simulink model "eVTOL_PX4_2023b"  (R2024b)
settings: Solver=ode4  StartTime=0  StopTime=inf  FixedStep=0.01  RelTol=1e-3
values from neighbouring files (symbols this model uses):
  aDl =     [initdata.mat]
  aDr =     [initdata.mat]
  aDyn =     [initdata.mat]
  Airport = init_airport('PHNL')    [initdata_HIL_eVTOL.m]
  aLat =     [initdata.mat]
  aLon =     [initdata.mat]
  D = Prop.D    [EOM_dt_MC.m]    (also in EOM_get_alf_dt_de_prop_evtol.m = CD * QS)
  dt0 = X(2)    [EOM_get_alf_dt_de_prop_evtol.m]    (also in initdata.mat = 0.258252593971; initdata_HIL_eVTOL.m = EOM_dt_MC)
  EAS0 = TAS0 / EAS2TAS    [initdata_HIL_eVTOL.m]
  FCS = init_FCS    [initdata_HIL_eVTOL.m]
  General = init_layoutdata    [EOM_dt_MC.m]    (also in build_optimized_CA.m; initdata.mat = ; initdata_HIL_eVTOL.m)
  h0 = Con(1)    [EOM_get_alf_dt_de_prop_evtol.m]    (also in initdata.mat = 450; initdata_HIL_eVTOL.m = 50)
  mass = Con(3)    [EOM_get_alf_dt_de_prop_evtol.m]    (also in initdata.mat = 2255.54; initdata_HIL_eVTOL.m = 7)
  Motor = init_motor_evtol    [EOM_dt_MC.m]    (also in initdata.mat = []; initdata_HIL_eVTOL.m)
  Prop = init_propeller_evtol_new    [EOM_dt_MC.m]    (also in initdata_HIL_eVTOL.m)
  R2D = 180/pi    (= 57.2957795131)    [EOM_get_alf_dt_de_prop_evtol.m]    (also in init_FCS.m; init_aerodata_evtol.m; init_airport.m; initdata.mat)
  SAMPLE_TIME = 0.01    [initdata_HIL_eVTOL.m]
  theta0 = -0.0510981441662    [initdata.mat]
undefined symbols (not defined in the file or in its folder): A1, aDa, aDe, aero, asbhl20env, B1, C1, de0, Earth, Environment, INIT_Data, InitData, Kd, Kp, magnitude, Newton, pProp, Raphson, Tc, WGS84
libraries: simulink_extras x63, vrlib x48, sharedtransform x28, simulink x22, slpidlib x20, sharedutil x20, matrix_library x18, aerolibwindfilters x12, aerolibobsolete x8, aerolibasang x8, aerolibatmos2 x6, aerolibfltsims x6
(part 15 of 17)

== system eVTOL_PX4_2023b/Subsystem1/Environment1/Wind Models/Dryden Wind Turbulence Model (Continuous (+q -r))/Select angular rates/Medium//High altitude rates ==
  pgw_h&l : Inport
  qgw_h&l : Inport  Port=2
  rgw_h&l : Inport  Port=3
  Action Port : ActionPort  PropagateVarSize=During execution  ActionPortLabel=elseif(u1>=min_height_high)
  Gain : Gain  SaturateOnIntegerOverflow=on  OutDataTypeStr=Inherit: Same as input  ParamDataTypeStr=Inherit: Same as input
  Mux : Mux  Inputs=3
  Selector3 : Selector  InputPortWidth=6  IndexOptions=Index vector (dialog)  Indices=[ 2 4 6]  OutputSizes=1
  pgw,qgw,rgw : Outport  InitialOutput=0  VectorParamsAs1DForOutWhenUnconnected=off
  wires:
  Gain/1 -> pgw,qgw,rgw/1
  Selector3/1 -> Gain/1
  pgw_h&l/1 -> Mux/1
  qgw_h&l/1 -> Mux/2
  rgw_h&l/1 -> Mux/3
  Mux/1 -> Selector3/1

== system eVTOL_PX4_2023b/Subsystem1/Environment1/Wind Models/Dryden Wind Turbulence Model (Continuous (+q -r))/Select angular rates/Merge Subsystems ==
  low : Inport
  high : Inport  Port=2
  interpolated : Inport  Port=3
  Demux : Demux  Outputs=3
      settings: DisplayOption=none
  Merge : Merge  Inputs=3
  pgw : Outport  VectorParamsAs1DForOutWhenUnconnected=off
  qgw : Outport  Port=2  VectorParamsAs1DForOutWhenUnconnected=off
  rgw : Outport  Port=3  VectorParamsAs1DForOutWhenUnconnected=off
  wires:
  low/1 -> Merge/1
  high/1 -> Merge/2
  interpolated/1 -> Merge/3
  Demux/2 -> qgw/1
  Demux/3 -> rgw/1
  Demux/1 -> pgw/1
  Merge/1 -> Demux/1

== system eVTOL_PX4_2023b/Subsystem1/Environment1/Wind Models/Dryden Wind Turbulence Model (Continuous (+q -r))/Select velocities/Interpolate velocities ==
  ugw_h&l : Inport
  vgw_h&l : Inport  Port=2
  wgw_h&l : Inport  Port=3
  DCM : Inport  Port=4
  Wind direction : Inport  Port=5
  Altitude : Inport  Port=6
  Action Port : ActionPort  PropagateVarSize=During execution  ActionPortLabel=else
  Mux : Mux  Inputs=3
  Mux1 : Mux  Inputs=3
  Product1 : Product  Inputs=**/  SaturateOnIntegerOverflow=on  OutDataTypeStr=Inherit: Same as first input
  Selector : Selector  InputPortWidth=2  IndexOptions=Index vector (dialog)  Indices=1  OutputSizes=1
  Selector1 : Selector  InputPortWidth=2  IndexOptions=Index vector (dialog)  Indices=1  OutputSizes=1
  Selector2 : Selector  InputPortWidth=2  IndexOptions=Index vector (dialog)  Indices=1  OutputSizes=1
  Selector3 : Selector  InputPortWidth=2  IndexOptions=Index vector (dialog)  Indices=2  OutputSizes=1
  Selector4 : Selector  InputPortWidth=2  IndexOptions=Index vector (dialog)  Indices=2  OutputSizes=1
  Selector5 : Selector  InputPortWidth=2  IndexOptions=Index vector (dialog)  Indices=2  OutputSizes=1
  Sum : Sum  Inputs=|-+  SaturateOnIntegerOverflow=on
  Sum1 : Sum  Inputs=|+-  SaturateOnIntegerOverflow=on
  Sum2 : Sum  Inputs=-+|  SaturateOnIntegerOverflow=on
  Sum3 : Sum  Inputs=++|  SaturateOnIntegerOverflow=on
  max_height_low : Constant  Value=max_height_low
  min_height_high : Constant  Value=min_height_high
  wind to body transformation : Subsystem
  ugw,vgw,wgw : Outport  InitialOutput=0  VectorParamsAs1DForOutWhenUnconnected=off
  wires:
  Mux/1 -> wind to body transformation/3(ug_l,vg_l,wg_l)
  Wind direction/1 -> wind to body transformation/2(Wind direction)
  DCM/1 -> wind to body transformation/1(DCM)
  wind to body transformation/1(ug,vg,wg) -> Sum3/1, Sum2/1
  Sum3/1 -> ugw,vgw,wgw/1
  Product1/1 -> Sum3/2
  Mux1/1 -> Sum2/2
  Sum2/1 -> Product1/1
  Sum1/1 -> Product1/2
  Sum/1 -> Product1/3
  Altitude/1 -> Sum1/1
  min_height_high/1 -> Sum/2
  max_height_low/1 -> Sum1/2, Sum/1
  Selector3/1 -> Mux1/1
  Selector4/1 -> Mux1/2
  Selector5/1 -> Mux1/3
  ugw_h&l/1 -> Selector/1, Selector3/1
  vgw_h&l/1 -> Selector4/1, Selector1/1
  wgw_h&l/1 -> Selector5/1, Selector2/1
  Selector/1 -> Mux/1
  Selector1/1 -> Mux/2
  Selector2/1 -> Mux/3

== system eVTOL_PX4_2023b/Subsystem1/Environment1/Wind Models/Dryden Wind Turbulence Model (Continuous (+q -r))/Select velocities/Low altitude velocities ==
  DCM : Inport
  ugw_h&l : Inport  Port=2
  vgw_h&l : Inport  Port=3
  wgw_h&l : Inport  Port=4
  Wind direction : Inport  Port=5
  Action Port : ActionPort  PropagateVarSize=During execution  ActionPortLabel=if(u1<=max_height_low)
  Mux : Mux  Inputs=3
  Selector : Selector  InputPortWidth=2  IndexOptions=Index vector (dialog)  Indices=1  OutputSizes=1
  Selector1 : Selector  InputPortWidth=2  IndexOptions=Index vector (dialog)  Indices=1  OutputSizes=1
  Selector2 : Selector  InputPortWidth=2  IndexOptions=Index vector (dialog)  Indices=1  OutputSizes=1
  wind to body transformation : Subsystem
  ugw,vgw,wgw : Outport  InitialOutput=0  VectorParamsAs1DForOutWhenUnconnected=off
  wires:
  Mux/1 -> wind to body transformation/3(ug_l,vg_l,wg_l)
  Selector2/1 -> Mux/3
  wind to body transformation/1(ug,vg,wg) -> ugw,vgw,wgw/1
  Wind direction/1 -> wind to body transformation/2(Wind direction)
  DCM/1 -> wind to body transformation/1(DCM)
  Selector1/1 -> Mux/2
  Selector/1 -> Mux/1
  wgw_h&l/1 -> Selector2/1
  vgw_h&l/1 -> Selector1/1
  ugw_h&l/1 -> Selector/1

== system eVTOL_PX4_2023b/Subsystem1/Environment1/Wind Models/Dryden Wind Turbulence Model (Continuous (+q -r))/Select velocities/Medium//High altitude velocities ==
  ugw_h&l : Inport
  vgw_h&l : Inport  Port=2
  wgw_h&l : Inport  Port=3
  Action Port : ActionPort  PropagateVarSize=During execution  ActionPortLabel=elseif(u1>=min_height_high)
  Gain : Gain  SaturateOnIntegerOverflow=on  OutDataTypeStr=Inherit: Same as input  ParamDataTypeStr=Inherit: Same as input
  Mux : Mux  Inputs=3
  Selector3 : Selector  InputPortWidth=6  IndexOptions=Index vector (dialog)  Indices=[ 2 4 6]  OutputSizes=1
  ugw,vgw,wgw : Outport  InitialOutput=0  VectorParamsAs1DForOutWhenUnconnected=off
  wires:
  vgw_h&l/1 -> Mux/2
  Gain/1 -> ugw,vgw,wgw/1
  Selector3/1 -> Gain/1
  Mux/1 -> Selector3/1
  wgw_h&l/1 -> Mux/3
  ugw_h&l/1 -> Mux/1

== system eVTOL_PX4_2023b/Subsystem1/Environment1/Wind Models/Dryden Wind Turbulence Model (Continuous (+q -r))/Select velocities/Merge Subsystems ==
  low : Inport
  high : Inport  Port=2
  interpolated : Inport  Port=3
  Demux : Demux  Outputs=3
      settings: DisplayOption=none
  Merge : Merge  Inputs=3
  ugw : Outport  VectorParamsAs1DForOutWhenUnconnected=off
  vgw : Outport  Port=2  VectorParamsAs1DForOutWhenUnconnected=off
  wgw : Outport  Port=3  VectorParamsAs1DForOutWhenUnconnected=off
  wires:
  Merge/1 -> Demux/1
  Demux/1 -> ugw/1
  Demux/3 -> wgw/1
  Demux/2 -> vgw/1
  interpolated/1 -> Merge/3
  high/1 -> Merge/2
  low/1 -> Merge/1

== system eVTOL_PX4_2023b/Subsystem1/Environment1/Wind Models/Dryden Wind Turbulence Model (Continuous (+q -r))/Turbulence scale lengths/Low altitude scale length ==
  h : Inport
  Limit Function 10ft to 1000ft : Saturate  UpperLimit=max_height_low  LowerLimit=10
  Low Altitude Scale Length : Fcn  Expr=u(1)/(0.177+0.000823*u(1))^1.2
  L_ug L_vg : Outport  InitialOutput=0  VectorParamsAs1DForOutWhenUnconnected=off
  L_wg : Outport  Port=2  InitialOutput=0  VectorParamsAs1DForOutWhenUnconnected=off
  wires:
  h/1 -> Limit Function 10ft to 1000ft/1
  Low Altitude Scale Length/1 -> L_ug L_vg/1
  Limit Function 10ft to 1000ft/1 -> L_wg/1, Low Altitude Scale Length/1

== system eVTOL_PX4_2023b/Subsystem1/Environment1/Wind Models/Dryden Wind Turbulence Model (Continuous (+q -r))/Turbulence scale lengths/Medium//High altitude scale length ==
  Length Conversion : Subsystem
  Medium/High Altitude : Constant  Value=L_high
  L_ug L_vg L_wg : Outport  Unit=ft  InitialOutput=0  VectorParamsAs1DForOutWhenUnconnected=off
  wires:
  Medium/High Altitude/1 -> Length Conversion/1(in)
  Length Conversion/1(out) -> L_ug L_vg L_wg/1

== system eVTOL_PX4_2023b/Subsystem1/airframe/force moment/aero F&M in body axis/Aerodynamic Coefficients/Actuator Increments ==
  Actuators : Inport
  incid : Inport  Port=2
  Aileron : Subsystem
  Bus Selector1 : BusSelector  OutputSignals=dl,dr,da
  Demux : Demux  Outputs=2
  Sum : Sum  Inputs=+++
  Terminator : Terminator
  V_left : Subsystem
  V_right : Subsystem
  cl : Outport  InitialOutput=0  VectorParamsAs1DForOutWhenUnconnected=off
  wires:
  Actuators/1 -> Bus Selector1/1
  Sum/1 -> cl/1
  V_right/1(dr_Coeff) -> Sum/2
  V_left/1(dl_Coeff) -> Sum/1
  Bus Selector1/1 -> V_left/2(dl)  "<dl>"
  Bus Selector1/3 -> Aileron/2(da)  "<da>"
  incid/1 -> Demux/1
  Demux/1 -> Aileron/1(alpha), V_right/1(alpha), V_left/1(alpha)  "alpha"
  Demux/2 -> Terminator/1  "beta"
  Aileron/1(da_Coeff) -> Sum/3
  Bus Selector1/2 -> V_right/2(dr)  "<dr>"

== system eVTOL_PX4_2023b/Subsystem1/airframe/force moment/aero F&M in body axis/Aerodynamic Coefficients/Basic Coefficients ==
  Incid : Inport
  mach : Inport  Port=2
  2-D Lookup Table : Lookup_n-D  NumberOfTableDimensions=1  BreakpointsForDimension1=aLon.alpha  BreakpointsForDimension2=aLon.mach  BreakpointsForDimension3=aLon.flap  Table=aLon.CL  InternalRulePriority=Speed  RndMeth=Simplest
  2-D Lookup Table1 : Lookup_n-D  NumberOfTableDimensions=1  BreakpointsForDimension1=aLon.alpha  BreakpointsForDimension2=aLon.mach  BreakpointsForDimension3=aLon.flap  Table=aLon.CD  InternalRulePriority=Speed  RndMeth=Simplest
  2-D Lookup Table2 : Lookup_n-D  NumberOfTableDimensions=1  BreakpointsForDimension1=aLon.alpha  BreakpointsForDimension2=aLon.mach  BreakpointsForDimension3=aLon.flap  Table=aLon.Cm  InternalRulePriority=Speed  RndMeth=Simplest
  2-D Lookup Table3 : Lookup_n-D  BreakpointsForDimension1=aLat.beta  BreakpointsForDimension2=aLat.alpha  BreakpointsForDimension3=aLat.mach  Table=aLat.dCD  InternalRulePriority=Speed  RndMeth=Simplest
      settings: InputPortMap=u0,u1
  2-D Lookup Table4 : Lookup_n-D  BreakpointsForDimension1=aLat.beta  BreakpointsForDimension2=aLat.alpha  BreakpointsForDimension3=aLat.mach  Table=aLat.dCY  InternalRulePriority=Speed  RndMeth=Simplest
      settings: InputPortMap=u0,u1
  2-D Lookup Table5 : Lookup_n-D  BreakpointsForDimension1=aLat.beta  BreakpointsForDimension2=aLat.alpha  BreakpointsForDimension3=aLat.mach  Table=aLat.dCl  InternalRulePriority=Speed  RndMeth=Simplest
      settings: InputPortMap=u0,u1
  2-D Lookup Table6 : Lookup_n-D  BreakpointsForDimension1=aLat.beta  BreakpointsForDimension2=aLat.alpha  BreakpointsForDimension3=aLat.mach  Table=aLat.dCL  InternalRulePriority=Speed  RndMeth=Simplest
      settings: InputPortMap=u0,u1
  2-D Lookup Table7 : Lookup_n-D  BreakpointsForDimension1=aLat.beta  BreakpointsForDimension2=aLat.alpha  BreakpointsForDimension3=aLat.mach  Table=aLat.dCm  InternalRulePriority=Speed  RndMeth=Simplest
      settings: InputPortMap=u0,u1
  2-D Lookup Table8 : Lookup_n-D  BreakpointsForDimension1=aLat.beta  BreakpointsForDimension2=aLat.alpha  BreakpointsForDimension3=aLat.mach  Table=aLat.dCn  InternalRulePriority=Speed  RndMeth=Simplest
      settings: InputPortMap=u0,u1
  Constant : Constant  Value=0
  Constant1 : Constant  Value=0
  Demux : Demux  Outputs=2
  Display : Display
  Display1 : Display
  Gain : Gain
  Mux1 : Mux  Inputs=6
  Mux2 : Mux  Inputs=6
  Saturation : Saturate  UpperLimit=0.1  LowerLimit=0
  Scope{1..5} (5 alike) : Scope
  Sum5 : Sum  Inputs=+++  InputSameDT=on  SaturateOnIntegerOverflow=on  OutDataTypeStr=Inherit: Same as first input
  "[-10,15]1" : Saturate  UpperLimit=15/57.3  LowerLimit=-10/57.3
  "[-15,15]" : Saturate  UpperLimit=15/57.3  LowerLimit=-15/57.3
  cl : Outport  InitialOutput=0  VectorParamsAs1DForOutWhenUnconnected=off
  wires:
  Mux1/1 -> Display/1, Sum5/2
  Demux/1 -> "[-10,15]1"/1  "alpha"
  Demux/2 -> "[-15,15]"/1  "beta"
  2-D Lookup Table1/1 -> Mux1/2, Scope3/1  "CD"
  Constant1/1 -> Mux1/6, Mux1/4, Mux1/3
  2-D Lookup Table4/1 -> Mux2/3  "dCY"
  2-D Lookup Table5/1 -> Mux2/4  "dCl"
  2-D Lookup Table8/1 -> Mux2/6  "dCn"
  Sum5/1 -> cl/1
  Mux2/1 -> Sum5/3, Display1/1
  Incid/1 -> Demux/1
  [alpha] -> 2-D Lookup Table/1, Scope4/1
  2-D Lookup Table/1 -> Scope2/1, Mux1/1  "CL"
  [alpha] -> 2-D Lookup Table1/1
  [alpha] -> 2-D Lookup Table2/1
  2-D Lookup Table2/1 -> Gain/1  "Cm"
  [beta] -> 2-D Lookup Table6/1
  2-D Lookup Table6/1 -> Mux2/1  "dCL"
  [alpha] -> 2-D Lookup Table6/2
  [alpha] -> 2-D Lookup Table3/2
  [beta] -> 2-D Lookup Table3/1
  2-D Lookup Table3/1 -> Mux2/2  "dCD"
  [beta] -> 2-D Lookup Table4/1
  [alpha] -> 2-D Lookup Table4/2
  [alpha] -> 2-D Lookup Table5/2
  [beta] -> 2-D Lookup Table5/1
  [beta] -> 2-D Lookup Table7/1
  [alpha] -> 2-D Lookup Table7/2
  2-D Lookup Table7/1 -> Mux2/5  "dCm"
  [alpha] -> 2-D Lookup Table8/2
  [beta] -> 2-D Lookup Table8/1
  Constant/1 -> Sum5/1
  Saturation/1 -> Scope1/1, [mach]
  mach/1 -> Saturation/1
  Gain/1 -> Mux1/5
  "[-15,15]"/1 -> [beta]
  "[-10,15]1"/1 -> Scope5/1, [alpha]

== system eVTOL_PX4_2023b/Subsystem1/airframe/force moment/aero F&M in body axis/Aerodynamic Coefficients/Body Rate Damping ==
  Incid : Inport
  pqrn : Inport  Port=2
  alphaDot_n : Inport  Port=3
  1-D Lookup Table : Lookup_n-D  NumberOfTableDimensions=1  BreakpointsForDimension1=aDyn.alpha  BreakpointsForDimension2=aDyn.flap  Table=aDyn.CYp  InternalRulePriority=Speed  RndMeth=Simplest
  1-D Lookup Table1 : Lookup_n-D  NumberOfTableDimensions=1  BreakpointsForDimension1=aDyn.alpha  BreakpointsForDimension2=aDyn.flap  Table=aDyn.Clp  InternalRulePriority=Speed  RndMeth=Simplest
  1-D Lookup Table2 : Lookup_n-D  NumberOfTableDimensions=1  BreakpointsForDimension1=aDyn.alpha  BreakpointsForDimension2=aDyn.flap  Table=aDyn.Cnp  InternalRulePriority=Speed  RndMeth=Simplest
  1-D Lookup Table3 : Lookup_n-D  NumberOfTableDimensions=1  BreakpointsForDimension1=aDyn.alpha  BreakpointsForDimension2=aDyn.flap  Table=aDyn.CYr  InternalRulePriority=Speed  RndMeth=Simplest
  1-D Lookup Table4 : Lookup_n-D  NumberOfTableDimensions=1  BreakpointsForDimension1=aDyn.alpha  BreakpointsForDimension2=aDyn.flap  Table=aDyn.Clr  InternalRulePriority=Speed  RndMeth=Simplest
  1-D Lookup Table5 : Lookup_n-D  NumberOfTableDimensions=1  BreakpointsForDimension1=aDyn.alpha  BreakpointsForDimension2=aDyn.flap  Table=aDyn.Cnr  InternalRulePriority=Speed  RndMeth=Simplest
  1-D Lookup Table6 : Lookup_n-D  NumberOfTableDimensions=1  BreakpointsForDimension1=aDyn.alpha  BreakpointsForDimension2=aDyn.flap  Table=aDyn.CLq  InternalRulePriority=Speed  RndMeth=Simplest
  1-D Lookup Table7 : Lookup_n-D  NumberOfTableDimensions=1  BreakpointsForDimension1=aDyn.alpha  BreakpointsForDimension2=aDyn.flap  Table=aDyn.Cmq  InternalRulePriority=Speed  RndMeth=Simplest
  1-D Lookup Table8 : Lookup_n-D  NumberOfTableDimensions=1  BreakpointsForDimension1=aDyn.alpha  BreakpointsForDimension2=aDyn.flap  Table=aDyn.CLAlphaDot  InternalRulePriority=Speed  RndMeth=Simplest
  1-D Lookup Table9 : Lookup_n-D  NumberOfTableDimensions=1  BreakpointsForDimension1=aDyn.alpha  BreakpointsForDimension2=aDyn.flap  Table=aDyn.CmAlphaDot  InternalRulePriority=Speed  RndMeth=Simplest
  Add : Sum  Inputs=++++
  Constant{,6..7,13} (4 alike) : Constant  Value=0
  Demux : Demux  Outputs=3
  Demux1 : Demux  Outputs=2
  Mux{1..4} (4 alike) : Mux  Inputs=6
  Product{4..7} (4 alike) : Product  InputSameDT=on  SaturateOnIntegerOverflow=on  OutDataTypeStr=Inherit: Same as first input
  Saturation : Saturate  UpperLimit=10/57.3  LowerLimit=-4/57.3
  Terminator : Terminator
  cl : Outport  InitialOutput=0  VectorParamsAs1DForOutWhenUnconnected=off
  wires:
  Add/1 -> cl/1
  1-D Lookup Table/1 -> Mux1/3  "CYp"
  1-D Lookup Table2/1 -> Mux1/6  "Cnp"
  Mux1/1 -> Product4/1
  1-D Lookup Table1/1 -> Mux1/4  "Clp"
  pqrn/1 -> Demux/1
  Demux/1 -> [p]
  Demux/2 -> [q]
  Demux/3 -> [r]
  Constant/1 -> Mux1/1, Mux1/2, Mux1/5
  1-D Lookup Table7/1 -> Mux2/5  "Cmq"
  1-D Lookup Table6/1 -> Mux2/1  "CLq"
  Mux2/1 -> Product5/1
  1-D Lookup Table3/1 -> Mux3/3  "CYr"
  Mux3/1 -> Product6/1
  1-D Lookup Table4/1 -> Mux3/4  "Clr"
  1-D Lookup Table5/1 -> Mux3/6  "Cnr"
  Constant7/1 -> Mux3/2, Mux3/5, Mux3/1
  Constant13/1 -> Mux4/6, Mux4/4, Mux4/3, Mux4/2
  1-D Lookup Table9/1 -> Mux4/5  "CmAlphaDot"
  1-D Lookup Table8/1 -> Mux4/1  "CLAlphaDot"
  Constant6/1 -> Mux2/4, Mux2/6, Mux2/3, Mux2/2
  [p] -> Product4/2
  [q] -> Product5/2
  [r] -> Product6/2
  Mux4/1 -> Product7/1
  alphaDot_n/1 -> Product7/2
  Product4/1 -> Add/1
  Product7/1 -> Add/4
  Demux1/2 -> Terminator/1  "beta"
  Demux1/1 -> [alpha]  "alpha"
  Incid/1 -> Demux1/1
  Product5/1 -> Add/3
  [alpha] -> Saturation/1
  Product6/1 -> Add/2
  Saturation/1 -> 1-D Lookup Table3/1, 1-D Lookup Table4/1, 1-D Lookup Table9/1, 1-D Lookup Table8/1, 1-D Lookup Table7/1, 1-D Lookup Table6/1, 1-D Lookup Table5/1, 1-D Lookup Table2/1, 1-D Lookup Table1/1, 1-D Lookup Table/1

== system eVTOL_PX4_2023b/Subsystem1/airframe/force moment/aero F&M in body axis/Aerodynamic Coefficients/CLCDCY-CXCYCZ ==
  Incid : Inport
  Cl_LDY : Inport  Port=2
  Cl_xA : Fcn  Expr=-u[4]*cos(u[2])*cos(u[1])+u[3]*sin(u[1])
  Cl_yA : Fcn  Expr=-u[4]*sin(u[2])+u[5]
  Cl_zA : Fcn  Expr=-u[4]*cos(u[2])*sin(u[1])-u[3]*cos(u[1])
  Mux : Mux  Inputs=3
  Mux1 : Mux  Inputs=2
  Cl_XYZ : Outport  VectorParamsAs1DForOutWhenUnconnected=off
  wires:
  Mux/1 -> Cl_XYZ/1
  Cl_LDY/1 -> Mux1/2
  Incid/1 -> Mux1/1
  Cl_zA/1 -> Mux/3
  Cl_yA/1 -> Mux/2
  Cl_xA/1 -> Mux/1
  Mux1/1 -> Cl_zA/1, Cl_yA/1, Cl_xA/1

== system eVTOL_PX4_2023b/Subsystem1/airframe1/force moment/aero F&M in body axis/Aerodynamic Coefficients/Actuator Increments ==
  Actuators : Inport
  incid : Inport  Port=2
  Aileron : Subsystem
  Bus Selector1 : BusSelector  OutputSignals=dl,dr,da
  Demux : Demux  Outputs=2
  Sum : Sum  Inputs=+++
  Terminator : Terminator
  V_left : Subsystem
  V_right : Subsystem
  cl : Outport  InitialOutput=0  VectorParamsAs1DForOutWhenUnconnected=off
  wires:
  Actuators/1 -> Bus Selector1/1
  Sum/1 -> cl/1
  V_right/1(dr_Coeff) -> Sum/2
  V_left/1(dl_Coeff) -> Sum/1
  Bus Selector1/1 -> V_left/2(dl)  "<dl>"
  Bus Selector1/3 -> Aileron/2(da)  "<da>"
  incid/1 -> Demux/1
  Demux/1 -> Aileron/1(alpha), V_right/1(alpha), V_left/1(alpha)  "alpha"
  Demux/2 -> Terminator/1  "beta"
  Aileron/1(da_Coeff) -> Sum/3
  Bus Selector1/2 -> V_right/2(dr)  "<dr>"

== system eVTOL_PX4_2023b/Subsystem1/airframe1/force moment/aero F&M in body axis/Aerodynamic Coefficients/Basic Coefficients ==
  Incid : Inport
  mach : Inport  Port=2
  2-D Lookup Table : Lookup_n-D  NumberOfTableDimensions=1  BreakpointsForDimension1=aLon.alpha  BreakpointsForDimension2=aLon.mach  BreakpointsForDimension3=aLon.flap  Table=aLon.CL  InternalRulePriority=Speed  RndMeth=Simplest
  2-D Lookup Table1 : Lookup_n-D  NumberOfTableDimensions=1  BreakpointsForDimension1=aLon.alpha  BreakpointsForDimension2=aLon.mach  BreakpointsForDimension3=aLon.flap  Table=aLon.CD  InternalRulePriority=Speed  RndMeth=Simplest
  2-D Lookup Table2 : Lookup_n-D  NumberOfTableDimensions=1  BreakpointsForDimension1=aLon.alpha  BreakpointsForDimension2=aLon.mach  BreakpointsForDimension3=aLon.flap  Table=aLon.Cm  InternalRulePriority=Speed  RndMeth=Simplest
  2-D Lookup Table3 : Lookup_n-D  BreakpointsForDimension1=aLat.beta  BreakpointsForDimension2=aLat.alpha  BreakpointsForDimension3=aLat.mach  Table=aLat.dCD  InternalRulePriority=Speed  RndMeth=Simplest
      settings: InputPortMap=u0,u1
  2-D Lookup Table4 : Lookup_n-D  BreakpointsForDimension1=aLat.beta  BreakpointsForDimension2=aLat.alpha  BreakpointsForDimension3=aLat.mach  Table=aLat.dCY  InternalRulePriority=Speed  RndMeth=Simplest
      settings: InputPortMap=u0,u1
  2-D Lookup Table5 : Lookup_n-D  BreakpointsForDimension1=aLat.beta  BreakpointsForDimension2=aLat.alpha  BreakpointsForDimension3=aLat.mach  Table=aLat.dCl  InternalRulePriority=Speed  RndMeth=Simplest
      settings: InputPortMap=u0,u1
  2-D Lookup Table6 : Lookup_n-D  BreakpointsForDimension1=aLat.beta  BreakpointsForDimension2=aLat.alpha  BreakpointsForDimension3=aLat.mach  Table=aLat.dCL  InternalRulePriority=Speed  RndMeth=Simplest
      settings: InputPortMap=u0,u1
  2-D Lookup Table7 : Lookup_n-D  BreakpointsForDimension1=aLat.beta  BreakpointsForDimension2=aLat.alpha  BreakpointsForDimension3=aLat.mach  Table=aLat.dCm  InternalRulePriority=Speed  RndMeth=Simplest
      settings: InputPortMap=u0,u1
  2-D Lookup Table8 : Lookup_n-D  BreakpointsForDimension1=aLat.beta  BreakpointsForDimension2=aLat.alpha  BreakpointsForDimension3=aLat.mach  Table=aLat.dCn  InternalRulePriority=Speed  RndMeth=Simplest
      settings: InputPortMap=u0,u1
  Constant : Constant  Value=0
  Constant1 : Constant  Value=0
  Demux : Demux  Outputs=2
  Display : Display
  Display1 : Display
  Gain : Gain
  Mux1 : Mux  Inputs=6
  Mux2 : Mux  Inputs=6
  Saturation : Saturate  UpperLimit=0.1  LowerLimit=0
  Scope{1..5} (5 alike) : Scope
  Sum5 : Sum  Inputs=+++  InputSameDT=on  SaturateOnIntegerOverflow=on  OutDataTypeStr=Inherit: Same as first input
  cl : Outport  InitialOutput=0  VectorParamsAs1DForOutWhenUnconnected=off
  wires:
  Mux1/1 -> Display/1, Sum5/2
  Demux/1 -> Scope5/1, [alpha]  "alpha"
  Demux/2 -> [beta]  "beta"
  2-D Lookup Table1/1 -> Mux1/2, Scope3/1  "CD"
  Constant1/1 -> Mux1/6, Mux1/4, Mux1/3
  2-D Lookup Table4/1 -> Mux2/3  "dCY"
  2-D Lookup Table5/1 -> Mux2/4  "dCl"
  2-D Lookup Table8/1 -> Mux2/6  "dCn"
  Sum5/1 -> cl/1
  Mux2/1 -> Sum5/3, Display1/1
  Incid/1 -> Demux/1
  [alpha] -> 2-D Lookup Table/1, Scope4/1
  2-D Lookup Table/1 -> Scope2/1, Mux1/1  "CL"
  [alpha] -> 2-D Lookup Table1/1
  [alpha] -> 2-D Lookup Table2/1
  2-D Lookup Table2/1 -> Gain/1  "Cm"
  [beta] -> 2-D Lookup Table6/1
  2-D Lookup Table6/1 -> Mux2/1  "dCL"
  [alpha] -> 2-D Lookup Table6/2
  [alpha] -> 2-D Lookup Table3/2
  [beta] -> 2-D Lookup Table3/1
  2-D Lookup Table3/1 -> Mux2/2  "dCD"
  [beta] -> 2-D Lookup Table4/1
  [alpha] -> 2-D Lookup Table4/2
  [alpha] -> 2-D Lookup Table5/2
  [beta] -> 2-D Lookup Table5/1
  [beta] -> 2-D Lookup Table7/1
  [alpha] -> 2-D Lookup Table7/2
  2-D Lookup Table7/1 -> Mux2/5  "dCm"
  [alpha] -> 2-D Lookup Table8/2
  [beta] -> 2-D Lookup Table8/1
  Constant/1 -> Sum5/1
  Saturation/1 -> Scope1/1, [mach]
  mach/1 -> Saturation/1
  Gain/1 -> Mux1/5

== system eVTOL_PX4_2023b/Subsystem1/airframe1/force moment/aero F&M in body axis/Aerodynamic Coefficients/Body Rate Damping ==
  Incid : Inport
  pqrn : Inport  Port=2
  alphaDot_n : Inport  Port=3
  1-D Lookup Table : Lookup_n-D  NumberOfTableDimensions=1  BreakpointsForDimension1=aDyn.alpha  BreakpointsForDimension2=aDyn.flap  Table=aDyn.CYp  InternalRulePriority=Speed  RndMeth=Simplest
  1-D Lookup Table1 : Lookup_n-D  NumberOfTableDimensions=1  BreakpointsForDimension1=aDyn.alpha  BreakpointsForDimension2=aDyn.flap  Table=aDyn.Clp  InternalRulePriority=Speed  RndMeth=Simplest
  1-D Lookup Table2 : Lookup_n-D  NumberOfTableDimensions=1  BreakpointsForDimension1=aDyn.alpha  BreakpointsForDimension2=aDyn.flap  Table=aDyn.Cnp  InternalRulePriority=Speed  RndMeth=Simplest
  1-D Lookup Table3 : Lookup_n-D  NumberOfTableDimensions=1  BreakpointsForDimension1=aDyn.alpha  BreakpointsForDimension2=aDyn.flap  Table=aDyn.CYr  InternalRulePriority=Speed  RndMeth=Simplest
  1-D Lookup Table4 : Lookup_n-D  NumberOfTableDimensions=1  BreakpointsForDimension1=aDyn.alpha  BreakpointsForDimension2=aDyn.flap  Table=aDyn.Clr  InternalRulePriority=Speed  RndMeth=Simplest
  1-D Lookup Table5 : Lookup_n-D  NumberOfTableDimensions=1  BreakpointsForDimension1=aDyn.alpha  BreakpointsForDimension2=aDyn.flap  Table=aDyn.Cnr  InternalRulePriority=Speed  RndMeth=Simplest
  1-D Lookup Table6 : Lookup_n-D  NumberOfTableDimensions=1  BreakpointsForDimension1=aDyn.alpha  BreakpointsForDimension2=aDyn.flap  Table=aDyn.CLq  InternalRulePriority=Speed  RndMeth=Simplest
  1-D Lookup Table7 : Lookup_n-D  NumberOfTableDimensions=1  BreakpointsForDimension1=aDyn.alpha  BreakpointsForDimension2=aDyn.flap  Table=aDyn.Cmq  InternalRulePriority=Speed  RndMeth=Simplest
  1-D Lookup Table8 : Lookup_n-D  NumberOfTableDimensions=1  BreakpointsForDimension1=aDyn.alpha  BreakpointsForDimension2=aDyn.flap  Table=aDyn.CLAlphaDot  InternalRulePriority=Speed  RndMeth=Simplest
  1-D Lookup Table9 : Lookup_n-D  NumberOfTableDimensions=1  BreakpointsForDimension1=aDyn.alpha  BreakpointsForDimension2=aDyn.flap  Table=aDyn.CmAlphaDot  InternalRulePriority=Speed  RndMeth=Simplest
  Add : Sum  Inputs=++++
  Constant{,6..7,13} (4 alike) : Constant  Value=0
  Demux : Demux  Outputs=3
  Demux1 : Demux  Outputs=2
  Mux{1..4} (4 alike) : Mux  Inputs=6
  Product{4..7} (4 alike) : Product  InputSameDT=on  SaturateOnIntegerOverflow=on  OutDataTypeStr=Inherit: Same as first input
  Terminator : Terminator
  cl : Outport  InitialOutput=0  VectorParamsAs1DForOutWhenUnconnected=off
  wires:
  Add/1 -> cl/1
  1-D Lookup Table/1 -> Mux1/3  "CYp"
  1-D Lookup Table2/1 -> Mux1/6  "Cnp"
  Mux1/1 -> Product4/1
  1-D Lookup Table1/1 -> Mux1/4  "Clp"
  pqrn/1 -> Demux/1
  Demux/1 -> [p]
  Demux/2 -> [q]
  Demux/3 -> [r]
  Constant/1 -> Mux1/1, Mux1/2, Mux1/5
  1-D Lookup Table7/1 -> Mux2/5  "Cmq"
  1-D Lookup Table6/1 -> Mux2/1  "CLq"
  Mux2/1 -> Product5/1
  1-D Lookup Table3/1 -> Mux3/3  "CYr"
  Mux3/1 -> Product6/1
  1-D Lookup Table4/1 -> Mux3/4  "Clr"
  1-D Lookup Table5/1 -> Mux3/6  "Cnr"
  Constant7/1 -> Mux3/2, Mux3/5, Mux3/1
  Constant13/1 -> Mux4/6, Mux4/4, Mux4/3, Mux4/2
  1-D Lookup Table9/1 -> Mux4/5  "CmAlphaDot"
  1-D Lookup Table8/1 -> Mux4/1  "CLAlphaDot"
  Constant6/1 -> Mux2/4, Mux2/6, Mux2/3, Mux2/2
  [p] -> Product4/2
  [q] -> Product5/2
  [r] -> Product6/2
  Mux4/1 -> Product7/1
  alphaDot_n/1 -> Product7/2
  Product4/1 -> Add/1
  Product7/1 -> Add/4
  Demux1/2 -> Terminator/1  "beta"
  Demux1/1 -> [alpha]  "alpha"
  Incid/1 -> Demux1/1
  Product5/1 -> Add/3
  [alpha] -> 1-D Lookup Table3/1, 1-D Lookup Table4/1, 1-D Lookup Table9/1, 1-D Lookup Table8/1, 1-D Lookup Table7/1, 1-D Lookup Table6/1, 1-D Lookup Table5/1, 1-D Lookup Table2/1, 1-D Lookup Table1/1, 1-D Lookup Table/1
  Product6/1 -> Add/2

== system eVTOL_PX4_2023b/Subsystem1/airframe1/force moment/aero F&M in body axis/Aerodynamic Coefficients/CLCDCY-CXCYCZ ==
  Incid : Inport
  Cl_LDY : Inport  Port=2
  Cl_xA : Fcn  Expr=-u[4]*cos(u[2])*cos(u[1])+u[3]*sin(u[1])
  Cl_yA : Fcn  Expr=-u[4]*sin(u[2])+u[5]
  Cl_zA : Fcn  Expr=-u[4]*cos(u[2])*sin(u[1])-u[3]*cos(u[1])
  Mux : Mux  Inputs=3
  Mux1 : Mux  Inputs=2
  Cl_XYZ : Outport  VectorParamsAs1DForOutWhenUnconnected=off
  wires:
  Mux/1 -> Cl_XYZ/1
  Cl_LDY/1 -> Mux1/2
  Incid/1 -> Mux1/1
  Cl_zA/1 -> Mux/3
  Cl_yA/1 -> Mux/2
  Cl_xA/1 -> Mux/1
  Mux1/1 -> Cl_zA/1, Cl_yA/1, Cl_xA/1

== system eVTOL_PX4_2023b/Subsystem2/Environment/Wind Models/Dryden Wind Turbulence Model (Continuous (+q -r))/RMS turbulence intensities/High Altitude Intensity ==
  h : Inport
  Medium/High Altitude Intensity : Interpolation_n-D  Table=sigma_vec'  ExtrapMethod=Clip  ValidIndexMayReachLast=on  OutDataTypeStr=double
  PreLook-Up Index Search (altitude) : PreLookup  BreakpointsData=h_vec  BeginIndexSearchUsingPreviousIndexResult=on  UseLastBreakpoint=on  FractionDataTypeStr=double
  PreLook-Up Index Search (prob of exceed) : PreLookup  BreakpointsData=[1:7]  BeginIndexSearchUsingPreviousIndexResult=on  UseLastBreakpoint=on  FractionDataTypeStr=double
  Probability of Exceedance : Constant  Value=TurbProb
  sigma_ug sigma_vg sigma_wg : Outport  InitialOutput=0  VectorParamsAs1DForOutWhenUnconnected=off
  wires:
  PreLook-Up Index Search (prob of exceed)/2 -> Medium/High Altitude Intensity/4
  PreLook-Up Index Search (prob of exceed)/1 -> Medium/High Altitude Intensity/3
  PreLook-Up Index Search (altitude)/2 -> Medium/High Altitude Intensity/2
  PreLook-Up Index Search (altitude)/1 -> Medium/High Altitude Intensity/1
  h/1 -> PreLook-Up Index Search (altitude)/1
  Medium/High Altitude Intensity/1 -> sigma_ug sigma_vg sigma_wg/1
  Probability of Exceedance/1 -> PreLook-Up Index Search (prob of exceed)/1

== system eVTOL_PX4_2023b/Subsystem2/Environment/Wind Models/Dryden Wind Turbulence Model (Continuous (+q -r))/RMS turbulence intensities/Low Altitude Intensity ==
  Windspeed at 20ft (6m) : Inport
  h : Inport  Port=2
  Limit Height h<1000ft : Saturate  UpperLimit=max_height_low  LowerLimit=0
  Low Altitude Intensity : Fcn  Expr=1/(0.177+0.000823*u(1))^0.4
  "sigma_ug, sigma_vg" : Product  InputSameDT=on  SaturateOnIntegerOverflow=on  OutDataTypeStr=Inherit: Same as first input
  "sigma_wg " : Gain  Gain=0.1  SaturateOnIntegerOverflow=on  OutDataTypeStr=Inherit: Same as input  ParamDataTypeStr=Inherit: Same as input
  sigma_ug sigma_vg : Outport  InitialOutput=0  VectorParamsAs1DForOutWhenUnconnected=off
  sigma_wg : Outport  Port=2  InitialOutput=0  VectorParamsAs1DForOutWhenUnconnected=off
  wires:
  "sigma_ug, sigma_vg"/1 -> sigma_ug sigma_vg/1
  h/1 -> Limit Height h<1000ft/1
  Low Altitude Intensity/1 -> "sigma_ug, sigma_vg"/1
  "sigma_wg "/1 -> sigma_wg/1, "sigma_ug, sigma_vg"/2
  Windspeed at 20ft (6m)/1 -> "sigma_wg "/1
  Limit Height h<1000ft/1 -> Low Altitude Intensity/1

== system eVTOL_PX4_2023b/Subsystem2/Environment/Wind Models/Dryden Wind Turbulence Model (Continuous (+q -r))/Select angular rates/Interpolate rates ==
  pgw_h&l : Inport
  qgw_h&l : Inport  Port=2
  rgw_h&l : Inport  Port=3
  DCM : Inport  Port=4
  Wind direction : Inport  Port=5
  Altitude : Inport  Port=6
  Action Port : ActionPort  PropagateVarSize=During execution  ActionPortLabel=else
  Mux : Mux  Inputs=3
  Mux1 : Mux  Inputs=3
  Product1 : Product  Inputs=**/  SaturateOnIntegerOverflow=on  OutDataTypeStr=Inherit: Same as first input
  Selector : Selector  InputPortWidth=2  IndexOptions=Index vector (dialog)  Indices=1  OutputSizes=1
  Selector1 : Selector  InputPortWidth=2  IndexOptions=Index vector (dialog)  Indices=1  OutputSizes=1
  Selector2 : Selector  InputPortWidth=2  IndexOptions=Index vector (dialog)  Indices=1  OutputSizes=1
  Selector3 : Selector  InputPortWidth=2  IndexOptions=Index vector (dialog)  Indices=2  OutputSizes=1
  Selector4 : Selector  InputPortWidth=2  IndexOptions=Index vector (dialog)  Indices=2  OutputSizes=1
  Selector5 : Selector  InputPortWidth=2  IndexOptions=Index vector (dialog)  Indices=2  OutputSizes=1
  Sum : Sum  Inputs=|-+  SaturateOnIntegerOverflow=on
  Sum1 : Sum  Inputs=|+-  SaturateOnIntegerOverflow=on
  Sum2 : Sum  Inputs=-+|  SaturateOnIntegerOverflow=on
  Sum3 : Sum  Inputs=++|  SaturateOnIntegerOverflow=on
  max_height_low : Constant  Value=max_height_low
  min_height_high : Constant  Value=min_height_high
  wind to body transformation : Subsystem
  pgw,qgw,rgw : Outport  InitialOutput=0  VectorParamsAs1DForOutWhenUnconnected=off
  wires:
  Mux/1 -> wind to body transformation/3(pg_l,qg_l,rg_l)
  DCM/1 -> wind to body transformation/1(DCM)
  wind to body transformation/1(pg,qg,rg) -> Sum3/1, Sum2/1
  Sum3/1 -> pgw,qgw,rgw/1
  Product1/1 -> Sum3/2
  Mux1/1 -> Sum2/2
  Sum2/1 -> Product1/1
  Sum1/1 -> Product1/2
  Sum/1 -> Product1/3
  Altitude/1 -> Sum1/1
  min_height_high/1 -> Sum/2
  max_height_low/1 -> Sum1/2, Sum/1
  Wind direction/1 -> wind to body transformation/2(Wind direction)
  Selector3/1 -> Mux1/1
  Selector4/1 -> Mux1/2
  Selector5/1 -> Mux1/3
  pgw_h&l/1 -> Selector/1, Selector3/1
  qgw_h&l/1 -> Selector4/1, Selector1/1
  rgw_h&l/1 -> Selector5/1, Selector2/1
  Selector/1 -> Mux/1
  Selector1/1 -> Mux/2
  Selector2/1 -> Mux/3

== system eVTOL_PX4_2023b/Subsystem2/Environment/Wind Models/Dryden Wind Turbulence Model (Continuous (+q -r))/Select angular rates/Low altitude rates ==
  DCM : Inport
  pgw_h&l : Inport  Port=2
  qgw_h&l : Inport  Port=3
  rgw_h&l : Inport  Port=4
  Wind direction : Inport  Port=5
  Action Port : ActionPort  PropagateVarSize=During execution  ActionPortLabel=if(u1<=max_height_low)
  Mux : Mux  Inputs=3
  Selector : Selector  InputPortWidth=2  IndexOptions=Index vector (dialog)  Indices=1  OutputSizes=1
  Selector1 : Selector  InputPortWidth=2  IndexOptions=Index vector (dialog)  Indices=1  OutputSizes=1
  Selector2 : Selector  InputPortWidth=2  IndexOptions=Index vector (dialog)  Indices=1  OutputSizes=1
  wind to body transformation : Subsystem
  pgw,qgw,rgw : Outport  InitialOutput=0  VectorParamsAs1DForOutWhenUnconnected=off
  wires:
  DCM/1 -> wind to body transformation/1(DCM)
  pgw_h&l/1 -> Selector/1
  qgw_h&l/1 -> Selector1/1
  rgw_h&l/1 -> Selector2/1
  Selector/1 -> Mux/1
  Selector1/1 -> Mux/2
  Selector2/1 -> Mux/3
  Mux/1 -> wind to body transformation/3(pg_l,qg_l,rg_l)
  wind to body transformation/1(pg,qg,rg) -> pgw,qgw,rgw/1
  Wind direction/1 -> wind to body transformation/2(Wind direction)

== system eVTOL_PX4_2023b/Subsystem2/Environment/Wind Models/Dryden Wind Turbulence Model (Continuous (+q -r))/Select angular rates/Medium//High altitude rates ==
  pgw_h&l : Inport
  qgw_h&l : Inport  Port=2
  rgw_h&l : Inport  Port=3
  Action Port : ActionPort  PropagateVarSize=During execution  ActionPortLabel=elseif(u1>=min_height_high)
  Gain : Gain  SaturateOnIntegerOverflow=on  OutDataTypeStr=Inherit: Same as input  ParamDataTypeStr=Inherit: Same as input
  Mux : Mux  Inputs=3
  Selector3 : Selector  InputPortWidth=6  IndexOptions=Index vector (dialog)  Indices=[ 2 4 6]  OutputSizes=1
  pgw,qgw,rgw : Outport  InitialOutput=0  VectorParamsAs1DForOutWhenUnconnected=off
  wires:
  Gain/1 -> pgw,qgw,rgw/1
  Selector3/1 -> Gain/1
  pgw_h&l/1 -> Mux/1
  qgw_h&l/1 -> Mux/2
  rgw_h&l/1 -> Mux/3
  Mux/1 -> Selector3/1

== system eVTOL_PX4_2023b/Subsystem2/Environment/Wind Models/Dryden Wind Turbulence Model (Continuous (+q -r))/Select angular rates/Merge Subsystems ==
  low : Inport
  high : Inport  Port=2
  interpolated : Inport  Port=3
  Demux : Demux  Outputs=3
      settings: DisplayOption=none
  Merge : Merge  Inputs=3
  pgw : Outport  VectorParamsAs1DForOutWhenUnconnected=off
  qgw : Outport  Port=2  VectorParamsAs1DForOutWhenUnconnected=off
  rgw : Outport  Port=3  VectorParamsAs1DForOutWhenUnconnected=off
  wires:
  low/1 -> Merge/1
  high/1 -> Merge/2
  interpolated/1 -> Merge/3
  Demux/2 -> qgw/1
  Demux/3 -> rgw/1
  Demux/1 -> pgw/1
  Merge/1 -> Demux/1

== system eVTOL_PX4_2023b/Subsystem2/Environment/Wind Models/Dryden Wind Turbulence Model (Continuous (+q -r))/Select velocities/Interpolate velocities ==
  ugw_h&l : Inport
  vgw_h&l : Inport  Port=2
  wgw_h&l : Inport  Port=3
  DCM : Inport  Port=4
  Wind direction : Inport  Port=5
  Altitude : Inport  Port=6
  Action Port : ActionPort  PropagateVarSize=During execution  ActionPortLabel=else
  Mux : Mux  Inputs=3
  Mux1 : Mux  Inputs=3
  Product1 : Product  Inputs=**/  SaturateOnIntegerOverflow=on  OutDataTypeStr=Inherit: Same as first input
  Selector : Selector  InputPortWidth=2  IndexOptions=Index vector (dialog)  Indices=1  OutputSizes=1
  Selector1 : Selector  InputPortWidth=2  IndexOptions=Index vector (dialog)  Indices=1  OutputSizes=1
  Selector2 : Selector  InputPortWidth=2  IndexOptions=Index vector (dialog)  Indices=1  OutputSizes=1
  Selector3 : Selector  InputPortWidth=2  IndexOptions=Index vector (dialog)  Indices=2  OutputSizes=1
  Selector4 : Selector  InputPortWidth=2  IndexOptions=Index vector (dialog)  Indices=2  OutputSizes=1
  Selector5 : Selector  InputPortWidth=2  IndexOptions=Index vector (dialog)  Indices=2  OutputSizes=1
  Sum : Sum  Inputs=|-+  SaturateOnIntegerOverflow=on
  Sum1 : Sum  Inputs=|+-  SaturateOnIntegerOverflow=on
  Sum2 : Sum  Inputs=-+|  SaturateOnIntegerOverflow=on
  Sum3 : Sum  Inputs=++|  SaturateOnIntegerOverflow=on
  max_height_low : Constant  Value=max_height_low
  min_height_high : Constant  Value=min_height_high
  wind to body transformation : Subsystem
  ugw,vgw,wgw : Outport  InitialOutput=0  VectorParamsAs1DForOutWhenUnconnected=off
  wires:
  Mux/1 -> wind to body transformation/3(ug_l,vg_l,wg_l)
  Wind direction/1 -> wind to body transformation/2(Wind direction)
  DCM/1 -> wind to body transformation/1(DCM)
  wind to body transformation/1(ug,vg,wg) -> Sum3/1, Sum2/1
  Sum3/1 -> ugw,vgw,wgw/1
  Product1/1 -> Sum3/2
  Mux1/1 -> Sum2/2
  Sum2/1 -> Product1/1
  Sum1/1 -> Product1/2
  Sum/1 -> Product1/3
  Altitude/1 -> Sum1/1
  min_height_high/1 -> Sum/2
  max_height_low/1 -> Sum1/2, Sum/1
  Selector3/1 -> Mux1/1
  Selector4/1 -> Mux1/2
  Selector5/1 -> Mux1/3
  ugw_h&l/1 -> Selector/1, Selector3/1
  vgw_h&l/1 -> Selector4/1, Selector1/1
  wgw_h&l/1 -> Selector5/1, Selector2/1
  Selector/1 -> Mux/1
  Selector1/1 -> Mux/2
  Selector2/1 -> Mux/3

== system eVTOL_PX4_2023b/Subsystem2/Environment/Wind Models/Dryden Wind Turbulence Model (Continuous (+q -r))/Select velocities/Low altitude velocities ==
  DCM : Inport
  ugw_h&l : Inport  Port=2
  vgw_h&l : Inport  Port=3
  wgw_h&l : Inport  Port=4
  Wind direction : Inport  Port=5
  Action Port : ActionPort  PropagateVarSize=During execution  ActionPortLabel=if(u1<=max_height_low)
  Mux : Mux  Inputs=3
  Selector : Selector  InputPortWidth=2  IndexOptions=Index vector (dialog)  Indices=1  OutputSizes=1
  Selector1 : Selector  InputPortWidth=2  IndexOptions=Index vector (dialog)  Indices=1  OutputSizes=1
  Selector2 : Selector  InputPortWidth=2  IndexOptions=Index vector (dialog)  Indices=1  OutputSizes=1
  wind to body transformation : Subsystem
  ugw,vgw,wgw : Outport  InitialOutput=0  VectorParamsAs1DForOutWhenUnconnected=off
  wires:
  Mux/1 -> wind to body transformation/3(ug_l,vg_l,wg_l)
  Selector2/1 -> Mux/3
  wind to body transformation/1(ug,vg,wg) -> ugw,vgw,wgw/1
  Wind direction/1 -> wind to body transformation/2(Wind direction)
  DCM/1 -> wind to body transformation/1(DCM)
  Selector1/1 -> Mux/2
  Selector/1 -> Mux/1
  wgw_h&l/1 -> Selector2/1
  vgw_h&l/1 -> Selector1/1
  ugw_h&l/1 -> Selector/1

== system eVTOL_PX4_2023b/Subsystem2/Environment/Wind Models/Dryden Wind Turbulence Model (Continuous (+q -r))/Select velocities/Medium//High altitude velocities ==
  ugw_h&l : Inport
  vgw_h&l : Inport  Port=2
  wgw_h&l : Inport  Port=3
  Action Port : ActionPort  PropagateVarSize=During execution  ActionPortLabel=elseif(u1>=min_height_high)
  Gain : Gain  SaturateOnIntegerOverflow=on  OutDataTypeStr=Inherit: Same as input  ParamDataTypeStr=Inherit: Same as input
  Mux : Mux  Inputs=3
  Selector3 : Selector  InputPortWidth=6  IndexOptions=Index vector (dialog)  Indices=[ 2 4 6]  OutputSizes=1
  ugw,vgw,wgw : Outport  InitialOutput=0  VectorParamsAs1DForOutWhenUnconnected=off
  wires:
  vgw_h&l/1 -> Mux/2
  Gain/1 -> ugw,vgw,wgw/1
  Selector3/1 -> Gain/1
  Mux/1 -> Selector3/1
  wgw_h&l/1 -> Mux/3
  ugw_h&l/1 -> Mux/1

== system eVTOL_PX4_2023b/Subsystem2/Environment/Wind Models/Dryden Wind Turbulence Model (Continuous (+q -r))/Select velocities/Merge Subsystems ==
  low : Inport
  high : Inport  Port=2
  interpolated : Inport  Port=3
  Demux : Demux  Outputs=3
      settings: DisplayOption=none
  Merge : Merge  Inputs=3
  ugw : Outport  VectorParamsAs1DForOutWhenUnconnected=off
  vgw : Outport  Port=2  VectorParamsAs1DForOutWhenUnconnected=off
  wgw : Outport  Port=3  VectorParamsAs1DForOutWhenUnconnected=off
  wires:
  Merge/1 -> Demux/1
  Demux/1 -> ugw/1
  Demux/3 -> wgw/1
  Demux/2 -> vgw/1
  interpolated/1 -> Merge/3
  high/1 -> Merge/2
  low/1 -> Merge/1

== system eVTOL_PX4_2023b/Subsystem2/Environment/Wind Models/Dryden Wind Turbulence Model (Continuous (+q -r))/Turbulence scale lengths/Low altitude scale length ==
  h : Inport
  Limit Function 10ft to 1000ft : Saturate  UpperLimit=max_height_low  LowerLimit=10
  Low Altitude Scale Length : Fcn  Expr=u(1)/(0.177+0.000823*u(1))^1.2
  L_ug L_vg : Outport  InitialOutput=0  VectorParamsAs1DForOutWhenUnconnected=off
  L_wg : Outport  Port=2  InitialOutput=0  VectorParamsAs1DForOutWhenUnconnected=off
  wires:
  h/1 -> Limit Function 10ft to 1000ft/1
  Low Altitude Scale Length/1 -> L_ug L_vg/1
  Limit Function 10ft to 1000ft/1 -> L_wg/1, Low Altitude Scale Length/1

== system eVTOL_PX4_2023b/Subsystem2/Environment/Wind Models/Dryden Wind Turbulence Model (Continuous (+q -r))/Turbulence scale lengths/Medium//High altitude scale length ==
  Length Conversion : Subsystem
  Medium/High Altitude : Constant  Value=L_high
  L_ug L_vg L_wg : Outport  Unit=ft  InitialOutput=0  VectorParamsAs1DForOutWhenUnconnected=off
  wires:
  Medium/High Altitude/1 -> Length Conversion/1(in)
  Length Conversion/1(out) -> L_ug L_vg L_wg/1

== system eVTOL_PX4_2023b/Subsystem2/airframe/force moment/aero F&M in body axis/Aerodynamic Coefficients/Actuator Increments ==
  Actuators : Inport
  incid : Inport  Port=2
  Aileron : Subsystem
  Bus Selector1 : BusSelector  OutputSignals=dl,dr,da
  Demux : Demux  Outputs=2
  Sum : Sum  Inputs=+++
  Terminator : Terminator
  V_left : Subsystem
  V_right : Subsystem
  cl : Outport  InitialOutput=0  VectorParamsAs1DForOutWhenUnconnected=off
  wires:
  Actuators/1 -> Bus Selector1/1
  Sum/1 -> cl/1
  V_right/1(dr_Coeff) -> Sum/2
  V_left/1(dl_Coeff) -> Sum/1
  Bus Selector1/1 -> V_left/2(dl)  "<dl>"
  Bus Selector1/3 -> Aileron/2(da)  "<da>"
  incid/1 -> Demux/1
  Demux/1 -> Aileron/1(alpha), V_right/1(alpha), V_left/1(alpha)  "alpha"
  Demux/2 -> Terminator/1  "beta"
  Aileron/1(da_Coeff) -> Sum/3
  Bus Selector1/2 -> V_right/2(dr)  "<dr>"

== system eVTOL_PX4_2023b/Subsystem2/airframe/force moment/aero F&M in body axis/Aerodynamic Coefficients/Basic Coefficients ==
  Incid : Inport
  mach : Inport  Port=2
  2-D Lookup Table : Lookup_n-D  NumberOfTableDimensions=1  BreakpointsForDimension1=aLon.alpha  BreakpointsForDimension2=aLon.mach  BreakpointsForDimension3=aLon.flap  Table=aLon.CL  InternalRulePriority=Speed  RndMeth=Simplest
  2-D Lookup Table1 : Lookup_n-D  NumberOfTableDimensions=1  BreakpointsForDimension1=aLon.alpha  BreakpointsForDimension2=aLon.mach  BreakpointsForDimension3=aLon.flap  Table=aLon.CD  InternalRulePriority=Speed  RndMeth=Simplest
  2-D Lookup Table2 : Lookup_n-D  NumberOfTableDimensions=1  BreakpointsForDimension1=aLon.alpha  BreakpointsForDimension2=aLon.mach  BreakpointsForDimension3=aLon.flap  Table=aLon.Cm  InternalRulePriority=Speed  RndMeth=Simplest
  2-D Lookup Table3 : Lookup_n-D  BreakpointsForDimension1=aLat.beta  BreakpointsForDimension2=aLat.alpha  BreakpointsForDimension3=aLat.mach  Table=aLat.dCD  InternalRulePriority=Speed  RndMeth=Simplest
      settings: InputPortMap=u0,u1
  2-D Lookup Table4 : Lookup_n-D  BreakpointsForDimension1=aLat.beta  BreakpointsForDimension2=aLat.alpha  BreakpointsForDimension3=aLat.mach  Table=aLat.dCY  InternalRulePriority=Speed  RndMeth=Simplest
      settings: InputPortMap=u0,u1
  2-D Lookup Table5 : Lookup_n-D  BreakpointsForDimension1=aLat.beta  BreakpointsForDimension2=aLat.alpha  BreakpointsForDimension3=aLat.mach  Table=aLat.dCl  InternalRulePriority=Speed  RndMeth=Simplest
      settings: InputPortMap=u0,u1
  2-D Lookup Table6 : Lookup_n-D  BreakpointsForDimension1=aLat.beta  BreakpointsForDimension2=aLat.alpha  BreakpointsForDimension3=aLat.mach  Table=aLat.dCL  InternalRulePriority=Speed  RndMeth=Simplest
      settings: InputPortMap=u0,u1
  2-D Lookup Table7 : Lookup_n-D  BreakpointsForDimension1=aLat.beta  BreakpointsForDimension2=aLat.alpha  BreakpointsForDimension3=aLat.mach  Table=aLat.dCm  InternalRulePriority=Speed  RndMeth=Simplest
      settings: InputPortMap=u0,u1
  2-D Lookup Table8 : Lookup_n-D  BreakpointsForDimension1=aLat.beta  BreakpointsForDimension2=aLat.alpha  BreakpointsForDimension3=aLat.mach  Table=aLat.dCn  InternalRulePriority=Speed  RndMeth=Simplest
      settings: InputPortMap=u0,u1
  Constant : Constant  Value=0
  Constant1 : Constant  Value=0
  Demux : Demux  Outputs=2
  Display : Display
  Display1 : Display
  Gain : Gain
  Mux1 : Mux  Inputs=6
  Mux2 : Mux  Inputs=6
  Saturation : Saturate  UpperLimit=0.1  LowerLimit=0
  Scope{1..5} (5 alike) : Scope
  Sum5 : Sum  Inputs=+++  InputSameDT=on  SaturateOnIntegerOverflow=on  OutDataTypeStr=Inherit: Same as first input
  cl : Outport  InitialOutput=0  VectorParamsAs1DForOutWhenUnconnected=off
  wires:
  Mux1/1 -> Display/1, Sum5/2
  Demux/1 -> Scope5/1, [alpha]  "alpha"
  Demux/2 -> [beta]  "beta"
  2-D Lookup Table1/1 -> Mux1/2, Scope3/1  "CD"
  Constant1/1 -> Mux1/6, Mux1/4, Mux1/3
  2-D Lookup Table4/1 -> Mux2/3  "dCY"
  2-D Lookup Table5/1 -> Mux2/4  "dCl"
  2-D Lookup Table8/1 -> Mux2/6  "dCn"
  Sum5/1 -> cl/1
  Mux2/1 -> Sum5/3, Display1/1
  Incid/1 -> Demux/1
  [alpha] -> 2-D Lookup Table/1, Scope4/1
  2-D Lookup Table/1 -> Scope2/1, Mux1/1  "CL"
  [alpha] -> 2-D Lookup Table1/1
  [alpha] -> 2-D Lookup Table2/1
  2-D Lookup Table2/1 -> Gain/1  "Cm"
  [beta] -> 2-D Lookup Table6/1
  2-D Lookup Table6/1 -> Mux2/1  "dCL"
  [alpha] -> 2-D Lookup Table6/2
  [alpha] -> 2-D Lookup Table3/2
  [beta] -> 2-D Lookup Table3/1
  2-D Lookup Table3/1 -> Mux2/2  "dCD"
  [beta] -> 2-D Lookup Table4/1
  [alpha] -> 2-D Lookup Table4/2
  [alpha] -> 2-D Lookup Table5/2
  [beta] -> 2-D Lookup Table5/1
  [beta] -> 2-D Lookup Table7/1
  [alpha] -> 2-D Lookup Table7/2
  2-D Lookup Table7/1 -> Mux2/5  "dCm"
  [alpha] -> 2-D Lookup Table8/2
  [beta] -> 2-D Lookup Table8/1
  Constant/1 -> Sum5/1
  Saturation/1 -> Scope1/1, [mach]
  mach/1 -> Saturation/1
  Gain/1 -> Mux1/5
